simulink model "RFB_parasitic_method"  (R2020a)
settings: Solver=VariableStepAuto  StartTime=0.0  StopTime=10.0  RelTol=1e-3
undefined symbols (not defined in the file): noise_bias, noise_power, relay_params
libraries: simulink x1, cstblocks x1
settings Model: Creator=rshousha  LastModifiedBy=jwai
settings DataIOCC: ReturnWorkspaceOutputs=off
settings DebuggingCC: ArithmeticOperatorsInVariantConditions=warning
settings SFSimCC: CustomCodeUndefinedFunction=UseInterfaceOnly

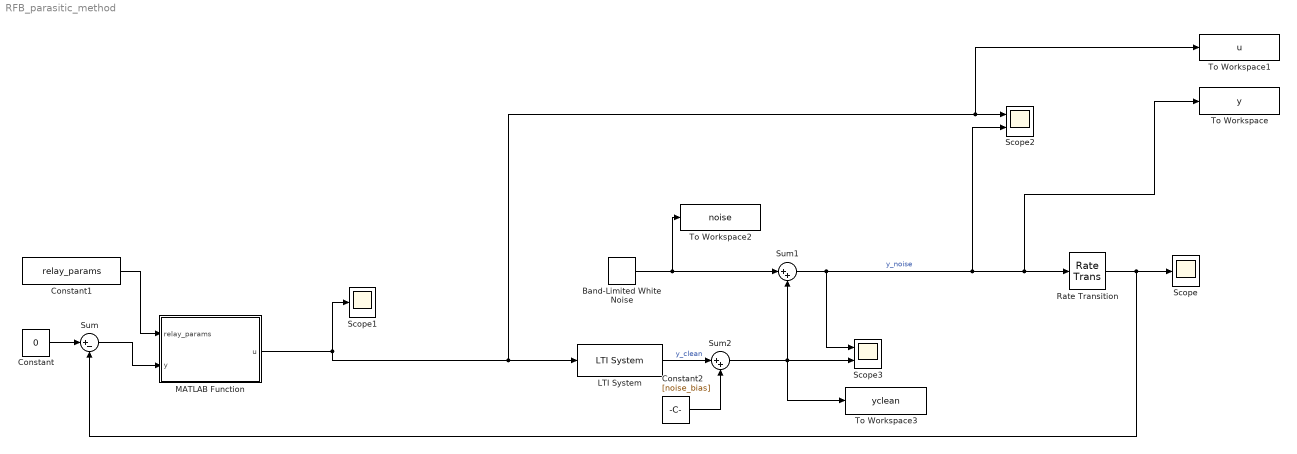
== system RFB_parasitic_method ==
  Band-Limited White Noise : simulink/Sources/Band-Limited White Noise  Cov=[noise_power]  Ts=5e-5  seed=[23341]
  Constant : Constant  Value=0
  Constant1 : Constant  Value=relay_params
  Constant2 : Constant  Value=[noise_bias]
  LTI System : cstblocks/LTI System  sys=G_true  IC=[]
  MATLAB Function : MATLAB Function  TreatAsAtomicUnit=on
  Rate Transition : RateTransition  OutPortSampleTime=5e-5
  Scope : Scope
  Scope1 : Scope
  Scope2 : Scope  NumInputPorts=2
  Scope3 : Scope  NumInputPorts=2
  Sum : Sum  Inputs=|+-
  Sum1 : Sum  Inputs=|++
  Sum2 : Sum  Inputs=|++
  To Workspace : ToWorkspace  VariableName=y  SaveFormat=Timeseries  SampleTime=-1
  To Workspace1 : ToWorkspace  VariableName=u  SaveFormat=Timeseries  SampleTime=-1
  To Workspace2 : ToWorkspace  VariableName=noise  SaveFormat=Timeseries  SampleTime=-1
  To Workspace3 : ToWorkspace  VariableName=yclean  SaveFormat=Timeseries  SampleTime=-1
  wires:
  Sum/1 -> MATLAB Function/2(y)
  Rate Transition/1 -> Scope/1, Sum/2
  Constant/1 -> Sum/1
  MATLAB Function/1(u) -> Scope1/1, To Workspace1/1, Scope2/1, LTI System/1
  Band-Limited White Noise/1 -> To Workspace2/1, Sum1/1
  Sum1/1 -> Scope3/1, Scope2/2, To Workspace/1, Rate Transition/1  "y_noise"
  Constant1/1 -> MATLAB Function/1(relay_params)
  LTI System/1 -> Sum2/1  "y_clean"
  Sum2/1 -> To Workspace3/1, Scope3/2, Sum1/2
  Constant2/1 -> Sum2/2

== matlab function RFB_parasitic_method/MATLAB Function ==
  data: relay_params input; y input; u output
function u  = parasitic_relay(relay_params, y)

persistent urelays_km1

d = relay_params(1);
output_bias_frac = relay_params(2);
input_bias = relay_params(3);
hysteresis = relay_params(4);
nparasites = relay_params(5);
alpha = relay_params(6:(5+nparasites));

beta = [1; alpha];  % multipliers for relays, including base relay

urelays = zeros(size(beta));
if isempty(urelays_km1)
  urelays = beta * d;
  urelays_km1 = urelays;
end

%% Base relay
if     (y > -input_bias + hysteresis)
    urelays(1) = d;
elseif (y < -input_bias - hysteresis)
    urelays(1) = -d;
else
    urelays(1) = urelays_km1(1);
end

%% Parasitic relays
for i = 2:length(beta)
  if (urelays_km1(i-1) > 0) && (urelays(i-1) < 0)
    urelays(i) = -beta(i) * abs(d) * sign(urelays_km1(i));
  else
    urelays(i) = urelays_km1(i);
  end
end

urelays_km1 = urelays;

%% Combined output with output bias
u = sum(urelays) + output_bias_frac * d;
    
    
end
